simulink model "autopilota_v_15_last"  (R2020b)
settings: Solver=ode4  StartTime=0.0  StopTime=300  FixedStep=0.02  RelTol=1e-3
values from neighbouring files (symbols this model uses):
  attuatore_Amax = 20*(pi/180)    (= 0.349065850399)    [v2021_10_27_avvioSITL.m]    (also in v2021_10_27_calcoloAerodinamica.m)
  attuatore_Amin = -20*(pi/180)    (= -0.349065850399)    [v2021_10_27_avvioSITL.m]
  attuatore_Emax = 25*(pi/180)    (= 0.436332312999)    [v2021_10_27_avvioSITL.m]    (also in v2021_10_27_calcoloAerodinamica.m)
  attuatore_Emin = -25*(pi/180)    (= -0.436332312999)    [v2021_10_27_avvioSITL.m]
  attuatore_Rmax = 25*(pi/180)    (= 0.436332312999)    [v2021_10_27_avvioSITL.m]    (also in v2021_10_27_calcoloAerodinamica.m)
  attuatore_Rmin = -25*(pi/180)    (= -0.436332312999)    [v2021_10_27_avvioSITL.m]
  attuatore_Tmax = 0.99    [v2021_10_27_avvioSITL.m]
  attuatore_Tmin = 0    [v2021_10_27_avvioSITL.m]
  bias = [baccxINI,baccyINI,bacczINI,bpINI,bqINI,brINI]    [v2021_10_27_avvioSITL.m]
  final_h = 35    [v2021_10_27_avvioSITL.m]
  interventoA_05 = 20*0.8    (= 16)    [v2021_10_27_avvioSITL.m]
  interventoA_1 = 10    [v2021_10_27_avvioSITL.m]
  interventoE_05 = 25*0.8    (= 20)    [v2021_10_27_avvioSITL.m]
  interventoE_1 = 10    [v2021_10_27_avvioSITL.m]
  interventoT = 1*0.6    (= 0.6)    [v2021_10_27_avvioSITL.m]
  inv_A = 1    [v2021_10_27_avvioSITL.m]
  inv_comp_h = 1    [v2021_10_27_avvioSITL.m]
  inv_E = 1    [v2021_10_27_avvioSITL.m]
  inv_R = 1    [v2021_10_27_avvioSITL.m]
  inv_T = 1    [v2021_10_27_avvioSITL.m]
  K_AW_B_AP_quota = 1000    [v2021_10_27_avvioSITL.m]
  K_AW_B_becc = -250    [v2021_10_27_avvioSITL.m]
  K_AW_B_imb = 0    [v2021_10_27_avvioSITL.m]
  K_AW_B_roll = 500    [v2021_10_27_avvioSITL.m]
  K_imb_inv = -0.001306    [v2021_10_27_avvioSITL.m]
  Kd_AP_rotta = 0.995    [v2021_10_27_avvioSITL.m]
  Kd_h_app = 0.085    [v2021_10_27_avvioSITL.m]
  Kd_h_flare = 0.01    [v2021_10_27_avvioSITL.m]
  Ki_AP_quota_select = 0.01936    [v2021_10_27_avvioSITL.m]
  Ki_AP_rotta = 0.002    [v2021_10_27_avvioSITL.m]
  Ki_AP_vel = 0.025175    [v2021_10_27_avvioSITL.m]
  Ki_becch = -0.1963    [v2021_10_27_avvioSITL.m]
  Ki_h_app = 0.055    [v2021_10_27_avvioSITL.m]
  Ki_h_cruise = 0.008    [v2021_10_27_avvioSITL.m]
  Ki_h_flare = 0.07    [v2021_10_27_avvioSITL.m]
  Ki_roll = 0.004528    [v2021_10_27_avvioSITL.m]
  Kp_AP_quota_hold_h = 0.5503    [v2021_10_27_avvioSITL.m]
  Kp_AP_quota_hold_l = 0.5503    [v2021_10_27_avvioSITL.m]
  Kp_AP_quota_select = 0.02647    [v2021_10_27_avvioSITL.m]
  Kp_AP_rotta = 0.520    (= 0.52)    [v2021_10_27_avvioSITL.m]
  Kp_AP_vel = 0.132175    [v2021_10_27_avvioSITL.m]
  Kp_becch = -0.30    (= -0.3)    [v2021_10_27_avvioSITL.m]
  Kp_comp_h = 0.035    [v2021_10_27_avvioSITL.m]
  Kp_h_app_max = 0.086    [v2021_10_27_avvioSITL.m]
  Kp_h_app_min = 0.01    [v2021_10_27_avvioSITL.m]
  Kp_h_cruise = 0.04    [v2021_10_27_avvioSITL.m]
  Kp_h_flare = 0.1    [v2021_10_27_avvioSITL.m]
  Kp_imb = 0.0019415    [v2021_10_27_avvioSITL.m]
  Kp_p = 0.006913    [v2021_10_27_avvioSITL.m]
  Kp_q = -0.025    [v2021_10_27_avvioSITL.m]
  Kp_roll = 0.0718    [v2021_10_27_avvioSITL.m]
  Kp_Rotta_ATO = 4    [v2021_10_27_avvioSITL.m]
  Kp_Rotta_psi = -0.01    [v2021_10_27_avvioSITL.m]
  Q1B = [    2e-15;     2e-15 ... (first row only)    [COV_F1B.m]
  R1B = [     2e-14;             2e-14 ... (first row only)    [COV_F1B.m]
  safe_phi = 55    [v2021_10_27_avvioSITL.m]
  safe_V = 40    [v2021_10_27_avvioSITL.m]
  Sensor_Offsets = [0,0,0]    [v2021_10_27_avvioSITL.m]
  T_cal = 0.4    [v2021_10_27_avvioSITL.m]
  theta_rot = 10    [v2021_10_27_avvioSITL.m]
  time_alarm_SAFE = 300    [v2021_10_27_avvioSITL.m]
  tsamp = 0.02    [v2021_10_27_avvioSITL.m]
  update = [2,2,2]    [v2021_10_27_avvioSITL.m]
  V_max = 35    [v2021_10_27_avvioSITL.m]
  V_stall = 15    [v2021_10_27_avvioSITL.m]
  vd_ini = 0    [v2021_10_27_avvioSITL.m]
  vel_wp1_al = 25    [v2021_10_27_avvioSITL.m]
  vel_wp2_al = 20    [v2021_10_27_avvioSITL.m]
undefined symbols (not defined in the file or in its folder): DiscIntNeverNeededParam, Newton, Raphson, t_AP
libraries: simulink_extras x41, pid_lib x8, dspsigops x4, simulink x3, aerolibtransform2sys x2, aerolibtransform2 x2, cstblocks x1, aerosimlib x1
(part 1 of 11)
settings Model: Creator=39339  LastModifiedBy=39334
settings DataIOCC: ReturnWorkspaceOutputs=off
settings DebuggingCC: ParameterPrecisionLossMsg=none  ArithmeticOperatorsInVariantConditions=warning
settings ModelReferenceCC: ModelReferenceNumInstancesAllowed=Single
settings SFSimCC: SimUseLocalCustomCode=off  CustomCodeUndefinedFunction=UseInterfaceOnly
settings RTWCC: RTWUseLocalCustomCode=off
settings CodeAppCC: StateflowObjectComments=on

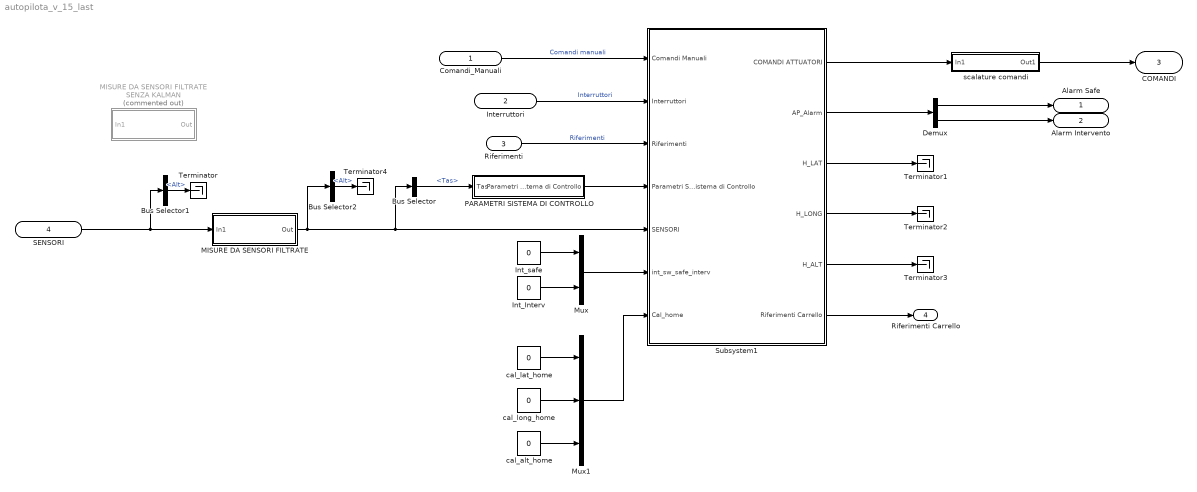
== system autopilota_v_15_last ==
  Comandi_Manuali : Inport  OutDataTypeStr=Bus: slBus4_manuali  SampleTime=[0.02,0]
  "Interruttori " : Inport  Port=2  OutDataTypeStr=Bus: slBus5_Interruttori  SampleTime=[0.02,0]
  Riferimenti : Inport  Port=3  OutDataTypeStr=Bus: slBus6_Riferimenti  SampleTime=[0.02,0]
  SENSORI : Inport  Port=4  OutDataTypeStr=Bus: slBus8_sensori2  SampleTime=[0.02,0]
  Bus Selector : BusSelector  OutputSignals=Tas
  Bus Selector1 : BusSelector  OutputSignals=Alt
  Bus Selector2 : BusSelector  OutputSignals=Alt
  Demux : Demux  Outputs=2
  Int_Interv : Constant  Value=0  SampleTime=t_AP
  Int_safe : Constant  Value=0  SampleTime=t_AP
  MISURE DA SENSORI FILTRATE : Subsystem
  MISURE DA SENSORI FILTRATE SENZA KALMAN : Subsystem  Commented=on
  Mux : Mux  Inputs=2
  Mux1 : Mux  Inputs=3
  PARAMETRI SISTEMA DI CONTROLLO : Subsystem
  Subsystem1 : Subsystem
  Terminator{,1..4} (5 alike) : Terminator
  cal_alt_home : Constant  Value=0  SampleTime=t_AP
  cal_lat_home : Constant  Value=0  SampleTime=t_AP
  cal_long_home : Constant  Value=0  SampleTime=t_AP
  "scalature comandi " : Subsystem
  Alarm Safe : Outport  OutDataTypeStr=double  PortDimensions=1  SampleTime=[0.02,0]  VectorParamsAs1DForOutWhenUnconnected=off
  Alarm Intervento : Outport  Port=2  OutDataTypeStr=double  PortDimensions=1  SampleTime=[0.02,0]  VectorParamsAs1DForOutWhenUnconnected=off
  "COMANDI " : Outport  Port=3  OutDataTypeStr=Bus: slBus8_comandi  SampleTime=[0.02,0]  VectorParamsAs1DForOutWhenUnconnected=off  LockScale=on
  Riferimenti Carrello : Outport  Port=4  VectorParamsAs1DForOutWhenUnconnected=off
  wires:
  cal_long_home/1 -> Mux1/2
  Comandi_Manuali/1 -> Subsystem1/1(Comandi Manuali)  "Comandi manuali"
  Bus Selector/1 -> PARAMETRI SISTEMA DI CONTROLLO/1(Tas)  "<Tas>"
  "Interruttori "/1 -> Subsystem1/2("Interruttori ")  "Interruttori"
  PARAMETRI SISTEMA DI CONTROLLO/1(Parametri Sistema di Controllo) -> Subsystem1/4(Parametri Sistema di Controllo)
  Subsystem1/3(H_LAT) -> Terminator1/1
  Demux/1 -> Alarm Safe/1
  Subsystem1/5(H_ALT) -> Terminator3/1
  cal_lat_home/1 -> Mux1/1
  Int_safe/1 -> Mux/1
  Riferimenti/1 -> Subsystem1/3(Riferimenti)  "Riferimenti"
  Mux1/1 -> Subsystem1/7(Cal_home)
  cal_alt_home/1 -> Mux1/3
  Int_Interv/1 -> Mux/2
  Demux/2 -> Alarm Intervento/1
  Subsystem1/4(H_LONG) -> Terminator2/1
  Subsystem1/2(AP_Alarm) -> Demux/1
  Mux/1 -> Subsystem1/6(int_sw_safe_interv)
  SENSORI/1 -> Bus Selector1/1, MISURE DA SENSORI FILTRATE/1(In1)
  MISURE DA SENSORI FILTRATE/1(Out) -> Bus Selector/1, Subsystem1/5(SENSORI), Bus Selector2/1
  "scalature comandi "/1(Out1) -> "COMANDI "/1
  Bus Selector2/1 -> Terminator4/1  "<Alt>"
  Bus Selector1/1 -> Terminator/1  "<Alt>"
  Subsystem1/6(Riferimenti Carrello) -> Riferimenti Carrello/1
  Subsystem1/1(COMANDI ATTUATORI) -> "scalature comandi "/1(In1)

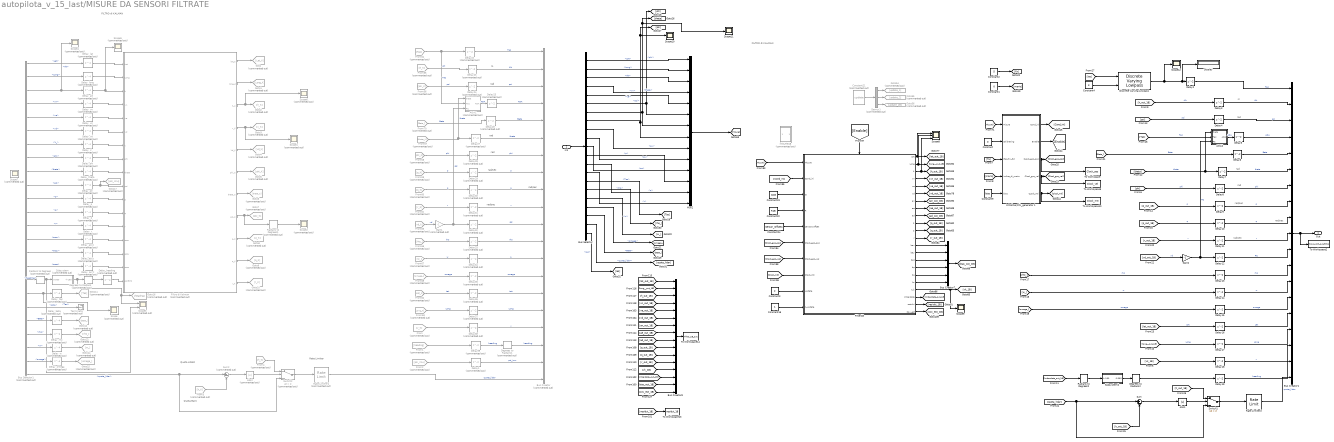
== system autopilota_v_15_last/MISURE DA SENSORI FILTRATE ==
  note: FILTRO di KALMAN
  note: m
  note: rad/sec
  note: rad/sec
  note: rad/sec
  note: rad
  note: rad
  note: rad
  note: Rate Limiter
  note: Quota Baro
  note: Quota LIDAR
  note: rad/sec
  note: rad/sec
  note: rad
  note: rad/sec
  note: FILTRO di KALMAN
  note: m
  note: rad
  note: rad
  In1 : Inport
  AOA1 : Subsystem  Commented=on
  AOA2 : Subsystem
  Abs1 : Abs
  Abs2 : Abs  Commented=on
  Bus Creator : BusCreator  Commented=on  Inputs=20  OutDataTypeStr=Bus: slBus7_sensori
  Bus Creator1 : BusCreator  Inputs=19  OutDataTypeStr=Bus: slBus7_sensori
  Bus Creator7 : BusCreator  Inputs=6
  Bus Creator8 : BusCreator  Inputs=16
  Bus Selector : BusSelector  OutputSignals=Lat,Long,Alt,vn,ve,phi,theta,psi,ax,ay,az,p,q,r,Tas,rho,w,omega,Beta,quota_lidar,Ias
  Bus Selector1 : BusSelector  Commented=on  OutputSignals=Lat,Long,Alt,vn,ve,vd,V_,phi,theta,psi,p,q,r,accx,accy,accz,heading,Tas,AOA,Beta,rho,w,omega,quota_lidar
  Constant : Constant  Value=0
  Constant1 : Constant  Value=0
  Constant16 : Constant
  Constant2 : Constant  Value=5
  Constant21 : Constant  Commented=on  Value=update
  Constant22 : Constant  Value=R1B
  Constant23 : Constant  Value=Q1B
  Constant24 : Constant  Value=Sensor_Offsets
  Constant3 : Constant  Value=2
  Constant4 : Constant  Value=3
  Constant9 : Constant  Value=bias
  Degrees to Radians : simulink_extras/Transformations/Degrees to Radians  Commented=on
  Degrees to Radians1 : simulink_extras/Transformations/Degrees to Radians  Commented=on
  Degrees to Radians2 : simulink_extras/Transformations/Degrees to Radians
  Delay{1,22..39} (19 alike) : Delay  Commented=on
  Delay{2..19} (18 alike) : Delay
  Delay_V_ : Delay  Commented=on  DelayLength=4
  Delay_accx : Delay  Commented=on  DelayLength=4
  Delay_accy : Delay  Commented=on  DelayLength=4
  Delay_accz : Delay  Commented=on  DelayLength=4
  Delay_alt : Delay  Commented=on  DelayLength=4
  Delay_beta : Delay  Commented=on  DelayLength=4
  Delay_heading : Delay  Commented=on  DelayLength=4
  Delay_lat : Delay  Commented=on  DelayLength=4
  Delay_long : Delay  Commented=on  DelayLength=4
  Delay_omega : Delay  Commented=on  DelayLength=4
  Delay_p : Delay  Commented=on  DelayLength=4
  Delay_phi : Delay  Commented=on  DelayLength=4
  Delay_psi : Delay  Commented=on  DelayLength=4
  Delay_q : Delay  Commented=on  DelayLength=4
  Delay_r : Delay  Commented=on  DelayLength=4
  Delay_rho : Delay  Commented=on  DelayLength=4
  Delay_tas : Delay  Commented=on  DelayLength=4
  Delay_theta : Delay  Commented=on  DelayLength=4
  Delay_vd : Delay  Commented=on  DelayLength=4
  Delay_ve : Delay  Commented=on  DelayLength=4
  Delay_vn : Delay  Commented=on  DelayLength=4
  Delay_w : Delay  Commented=on  DelayLength=4
  Demux1 : Demux  Commented=on  Outputs=3
  Discrete Varying Lowpass : cstblocks/Linear Parameter Varying/Discrete Varying Lowpass  N=2  w0=0  Ts=0.02
      settings: SourceProductBaseCode=CT
  Display : Display
  Filter1B : Subsystem
  Filtro di Kalman : Subsystem  Commented=on
  From : From  Commented=on  GotoTag=v_K
  From1 : From  Commented=on  GotoTag=heading
  From2 : From  Commented=on  GotoTag=psi_imu
  From3 : From  Commented=on  GotoTag=h_K
  From4 : From  Commented=on  GotoTag=h_K
  From55 : From  Commented=on  GotoTag=h_K
  From56 : From  Commented=on  GotoTag=psi_K
  From57 : From  Commented=on  GotoTag=theta_K
  From58 : From  Commented=on  GotoTag=phi_K
  From59 : From  Commented=on  GotoTag=p_K
  From60 : From  Commented=on  GotoTag=q_K
  From61 : From  Commented=on  GotoTag=r_K
  From62 : From  Commented=on  GotoTag=Lat_K
  From63 : From  Commented=on  GotoTag=Long_K
  From64 : From  Commented=on  GotoTag=Tas
  From65 : From  Commented=on  GotoTag=vd_k
  From66 : From  Commented=on  GotoTag=rho_
  From67 : From  Commented=on  GotoTag=w_
  From68 : From  Commented=on  GotoTag=omega_
  From70 : From  Commented=on  GotoTag=Beta_
  Gain1 : Gain  Commented=on  Gain=-1
  Gain2 : Gain  Gain=-1
  Goto : Goto  Commented=on  GotoTag=Lat_K
  Goto1 : Goto  Commented=on  GotoTag=Long_K
  Goto10 : Goto  Commented=on  GotoTag=r_K
  Goto11 : Goto  Commented=on  GotoTag=Tas
  Goto12 : Goto  Commented=on  GotoTag=Beta_
  Goto13 : Goto  Commented=on  GotoTag=rho_
  Goto14 : Goto  Commented=on  GotoTag=w_
  Goto15 : Goto  Commented=on  GotoTag=omega_
  Goto16 : Goto  Commented=on  GotoTag=heading
  Goto17 : Goto  Commented=on  GotoTag=psi_imu
  Goto2 : Goto  Commented=on  GotoTag=h_K
  Goto3 : Goto  Commented=on  GotoTag=v_K
  Goto4 : Goto  Commented=on  GotoTag=vd_k
  Goto5 : Goto  Commented=on  GotoTag=phi_K
  Goto54 : Goto  Commented=on  GotoTag=update_1
  Goto55 : Goto  Commented=on  GotoTag=update_2
  Goto56 : Goto  Commented=on  GotoTag=update_2B
  Goto6 : Goto  Commented=on  GotoTag=theta_K
  Goto7 : Goto  Commented=on  GotoTag=psi_K
  Goto8 : Goto  Commented=on  GotoTag=p_K
  Goto9 : Goto  Commented=on  GotoTag=q_K
  MISURE1B : Subsystem  Commented=on
  Mux2 : Mux  Inputs=14
  Radians to Degrees : simulink_extras/Transformations/Radians to Degrees  Commented=on
  Radians to Degrees1 : simulink_extras/Transformations/Radians to Degrees  Commented=on
  Radians to Degrees2 : simulink_extras/Transformations/Radians to Degrees
  Rate Limiter1 : RateLimiter  Commented=on  RisingSlewLimit=6  FallingSlewLimit=-6  SampleTimeMode=inherited
  Rate Limiter2 : RateLimiter  RisingSlewLimit=6  FallingSlewLimit=-6  SampleTimeMode=inherited
  Scope{,1..2,4..7} (7 alike) : Scope  Commented=on
  Scope{9..12} (4 alike) : Scope
  Scope3 : Scope  Commented=on  NumInputPorts=2
  Scope8 : Scope  NumInputPorts=3
  Subsystem : Subsystem  Commented=on
  Subsystem2 : Subsystem
  Sum : Sum  Inputs=|+-
  Sum2 : Sum  Commented=on  Inputs=|+-
  Switch1 : Switch  Criteria=u2 > Threshold  Threshold=2
  Switch2 : Switch  Commented=on  Criteria=u2 > Threshold  Threshold=2
  Terminator : Terminator  Commented=on
  To Workspace : ToWorkspace  VariableName=Clock_pos  SaveFormat=Timeseries  SampleTime=-1
  To Workspace10 : ToWorkspace  VariableName=Clock_mti  SaveFormat=Timeseries  SampleTime=-1
  To Workspace13 : ToWorkspace  VariableName=residui_1B  SaveFormat=Structure With Time  SampleTime=-1
  To Workspace14 : ToWorkspace  VariableName=Filtro_1B_out  SaveFormat=Timeseries  SampleTime=-1
  To Workspace2 : ToWorkspace  VariableName=Prova_WP_out_filtro  SaveFormat=Timeseries  SampleTime=-1
  To Workspace9 : ToWorkspace  VariableName=Clock_vel  SaveFormat=Timeseries  SampleTime=-1
  initializer/Clk_generator 1 : Subsystem
  Out : Outport  OutDataTypeStr=Bus: slBus7_sensori  VectorParamsAs1DForOutWhenUnconnected=off
  wires:
  Bus Selector1/1 -> Delay_lat/1  "<Lat>"
  Bus Selector1/23 -> Delay_omega/1  "<omega>"
  Bus Selector1/2 -> Delay_long/1  "<Long>"
  Bus Selector1/3 -> Scope4/1, Delay_alt/1  "<Alt>"
  Bus Selector1/4 -> Delay_vn/1  "<vn>"
  Bus Selector1/5 -> Delay_ve/1  "<ve>"
  Bus Selector1/6 -> Delay_vd/1  "<vd>"
  Bus Selector1/7 -> Delay_V_/1  "<V_>"
  Bus Selector1/8 -> Delay_phi/1  "<phi>"
  Bus Selector1/9 -> Delay_theta/1  "<theta>"
  Bus Selector1/10 -> Delay_psi/1  "<psi>"
  Bus Selector1/11 -> Delay_p/1  "<p>"
  Bus Selector1/12 -> Delay_q/1  "<q>"
  Bus Selector1/13 -> Delay_r/1  "<r>"
  Bus Selector1/14 -> Delay_accx/1  "<accx>"
  Bus Selector1/15 -> Delay_accy/1  "<accy>"
  Bus Selector1/16 -> Delay_accz/1  "<accz>"
  Bus Selector1/17 -> Radians to Degrees/1  "<heading>"
  Filtro di Kalman/1(lat_K) -> Goto/1
  Filtro di Kalman/2(long_K) -> Goto1/1
  Filtro di Kalman/3(h_K) -> Scope6/1, Goto2/1
  Filtro di Kalman/4(v_K) -> Scope1/1, Goto3/1
  Filtro di Kalman/6(phi_K) -> Goto5/1
  Filtro di Kalman/7(theta_K) -> Goto6/1
  Filtro di Kalman/9(p_K) -> Goto8/1
  Filtro di Kalman/11(r_K) -> Goto10/1
  Filtro di Kalman/10(q_K) -> Goto9/1
  Bus Selector1/18 -> Scope/1, Delay_tas/1  "<Tas>"
  Bus Selector1/19 -> Terminator/1  "<AOA>"
  Bus Selector1/20 -> Delay_beta/1  "<Beta>"
  Bus Selector1/21 -> Delay_rho/1  "<rho>"
  Bus Selector1/22 -> Delay_w/1  "<w>"
  From55/1 -> Delay23/1  "Alt"
  From56/1 -> Delay24/1  "psi"
  From57/1 -> AOA1/1(theta), Delay27/1  "theta"
  From58/1 -> Delay28/1  "phi"
  From59/1 -> Delay29/1  "p"
  From60/1 -> Delay30/1  "q"
  From61/1 -> Delay31/1  "r"
  From63/1 -> Delay37/1  "Long"
  From64/1 -> AOA1/2(Tas), Delay22/1  "Tas"
  From65/1 -> Gain1/1  "vd"
  From66/1 -> Delay33/1  "rho"
  From67/1 -> Delay34/1  "w"
  From68/1 -> Delay35/1  "omega"
  AOA1/1(AOA) -> Delay25/1  "AOA"
  From70/1 -> Delay26/1  "Beta"
  From62/1 -> Delay36/1  "Lat"
  Gain1/1 -> AOA1/3(RC), Delay32/1  "RC"
  Filtro di Kalman/5(Vd_K) -> Goto4/1
  Delay_lat/1 -> Filtro di Kalman/1("Lat ")
  Delay_long/1 -> Filtro di Kalman/2("Long ")
  Delay_psi/1 -> Goto17/1, Filtro di Kalman/10(psi)
  Delay_p/1 -> Filtro di Kalman/11(p)
  Delay_q/1 -> Filtro di Kalman/12(q)
  Delay_r/1 -> Filtro di Kalman/13(r)
  Delay_accx/1 -> Filtro di Kalman/14(accx)
  Delay_accy/1 -> Filtro di Kalman/15(accy)
  Delay_accz/1 -> Filtro di Kalman/16(accz)
  Delay_vd/1 -> Filtro di Kalman/6(vd)
  Delay_V_/1 -> Filtro di Kalman/7("v ")
  Delay_theta/1 -> Filtro di Kalman/9(theta)
  Delay_ve/1 -> Filtro di Kalman/5("ve ")
  Delay_vn/1 -> Filtro di Kalman/4(vn)
  Delay_alt/1 -> Scope5/1, Filtro di Kalman/3(h)
  Delay_phi/1 -> Filtro di Kalman/8(phi)
  Delay_tas/1 -> Goto11/1
  Delay_beta/1 -> Goto12/1
  Delay_rho/1 -> Goto13/1
  Delay_w/1 -> Goto14/1
  Delay_omega/1 -> Goto15/1
  Filtro di Kalman/8(psi_K) -> Radians to Degrees1/1, Goto7/1
  Radians to Degrees1/1 -> Scope2/1
  Delay22/1 -> Bus Creator/1  "Tas"
  Delay23/1 -> Bus Creator/2  "Alt"
  Delay24/1 -> Bus Creator/3  "psi"
  Delay25/1 -> Bus Creator/4  "AOA"
  Delay26/1 -> Bus Creator/5  "Beta"
  Delay27/1 -> Bus Creator/6  "theta"
  Delay28/1 -> Bus Creator/7  "phi"
  Delay29/1 -> Bus Creator/8  "p"
  Delay30/1 -> Bus Creator/9  "q"
  Delay31/1 -> Bus Creator/10  "r"
  Delay32/1 -> Bus Creator/11  "RC"
  Delay33/1 -> Bus Creator/12  "rho"
  Delay34/1 -> Bus Creator/13  "w"
  Delay35/1 -> Bus Creator/14  "omega"
  Delay36/1 -> Bus Creator/15  "Lat"
  Delay37/1 -> Bus Creator/16  "Long"
  Subsystem/1("+-180 ") -> Degrees to Radians/1, Scope3/1, Goto16/1
  Radians to Degrees/1 -> Scope3/2, Subsystem/1(0-360)
  Delay_heading/1 -> Filtro di Kalman/17(psiGPS)
  Degrees to Radians/1 -> Delay_heading/1
  Delay38/1 -> Bus Creator/17  "v"
  From/1 -> Delay38/1
  From1/1 -> Delay39/1
  Delay39/1 -> Degrees to Radians1/1  "heading"
  From2/1 -> Delay1/1
  Delay1/1 -> Bus Creator/19  "psi_imu"
  Bus Selector1/24 -> Switch2/3, Sum2/1  "<quota_lidar>"
  Abs2/1 -> Switch2/2
  Switch2/1 -> Rate Limiter1/1
  From3/1 -> Sum2/2
  From4/1 -> Switch2/1
  Rate Limiter1/1 -> Bus Creator/20  "quota_lidar"
  Sum2/1 -> Abs2/1
  Degrees to Radians1/1 -> Bus Creator/18  "heading"
  Constant16/1 -> Filter1B/10(k_update)
  [Misure] -> initializer/Clk_generator 1/1(Misure)
  Delay14/1 -> Bus Creator1/13  "w"
  [Clock_gps_vel] -> Filter1B/7(Clock_gps_vel)
  Filter1B/21(residui) -> [residui_1B]
  Bus Selector/14 -> Mux2/14  "<r>"
  Filter1B/11(q) -> [q_out_1B]
  Filter1B/9(ad) -> [ad_out_1B]
  Filter1B/16(bp) -> Bus Creator7/4
  Gain2/1 -> AOA2/3(RC), Delay12/1  "RC"
  Filter1B/17(bq) -> Bus Creator7/5
  [long__out_1B] -> Bus Creator8/2
  [Clock_mti] -> Filter1B/8(Clock_mti)
  [mario] -> initializer/Clk_generator 1/4(indice_di_mario)
  Bus Creator7/1 -> [bias_out_1B]
  [h_out_1B] -> Bus Creator8/3
  [an_out_1B] -> Bus Creator8/7
  [Clock_gps_pos] -> Filter1B/6(Clock_gps_pos)
  Bus Selector/10 -> Mux2/10  "<ay>"
  [ad_out_1B] -> Bus Creator8/9
  Filter1B/5(ve) -> [ve_out_1B]
  Filter1B/3(h) -> Scope8/3, [h_out_1B]
  [ae_out_1B] -> Bus Creator8/8
  Bus Creator8/1 -> To Workspace14/1
  Bus Selector/13 -> Mux2/13  "<q>"
  Constant3/1 -> Filter1B/9(update)
  [h_out_1B] -> Delay3/1  "Alt"
  Constant9/1 -> initializer/Clk_generator 1/5(bias)
  Filter1B/4(vn) -> [vn_out_1B]
  [lat_out_1B] -> Delay16/1  "Lat"
  [w_] -> Delay14/1  "w"
  Constant24/1 -> Filter1B/5(sensors offset)
  [Cond_ini] -> Filter1B/2(Cond_ini)
  Constant2/1 -> [fix]
  Filter1B/13(bax) -> Bus Creator7/1
  Filter1B/8(ae) -> [ae_out_1B]
  Filter1B/15(baz) -> Bus Creator7/3
  Delay19/1 -> Bus Creator1/18  "heading"
  [Misure] -> Filter1B/1(Misure)
  Delay9/1 -> Bus Creator1/8  "p"
  Filter1B/12(r) -> [r_out_1B]
  [vd_out_1B] -> Gain2/1  "vd"
  Filter1B/10(p) -> [p_out_1B]
  [cov_est_1B] -> Bus Creator8/16
  initializer/Clk_generator 1/5(CLock_mti) -> To Workspace10/1, [Clock_mti]
  Filter1B/6(vd) -> [vd_out_1B]
  Filter1B/22(Cov_est) -> [cov_est_1B]
  [vk_1B] -> Delay18/1
  initializer/Clk_generator 1/2(Enable) -> [Enable]
  [vn_out_1B] -> Bus Creator8/4
  [imbardata_out_1B] -> Bus Creator8/14
  [vd_out_1B] -> Bus Creator8/6
  [Beta_] -> Delay6/1  "Beta"
  Delay6/1 -> Bus Creator1/5  "Beta"
  [rho_] -> Delay13/1  "rho"
  Demux1/2 -> Goto55/1
  Mux2/1 -> [Misure]
  Demux1/1 -> Goto54/1
  initializer/Clk_generator 1/4("Clock_gps_vel ") -> To Workspace9/1, [Clock_gps_vel]
  Delay4/1 -> Bus Creator1/3  "psi"
  [bias_out_1B] -> Bus Creator8/15
  Filter1B/18(br) -> Bus Creator7/6
  [ve_out_1B] -> Bus Creator8/5
  Constant/1 -> initializer/Clk_generator 1/2(calibrating)
  initializer/Clk_generator 1/3(CLock_gps_pos) -> To Workspace/1, [Clock_gps_pos]
  Delay15/1 -> Bus Creator1/14  "omega"
  Constant22/1 -> Filter1B/4(R)
  [p_out_1B] -> Delay9/1  "p"
  [phi] -> Delay8/1  "phi"
  Filter1B/2(Long) -> [long__out_1B], Scope8/2
  Bus Selector/5 -> Mux2/5  "<ve>"
  [lat_out_1B] -> Bus Creator8/1
  Bus Selector/15 -> [Tas]  "<Tas>"
  Delay18/1 -> Bus Creator1/17  "v"
  [q_out_1B] -> Bus Creator8/11
  Bus Selector/1 -> Mux2/1  "<Lat>"
  initializer/Clk_generator 1/1(Cond_ini) -> [Cond_ini]
  [fix] -> initializer/Clk_generator 1/3(Gps_fix_3d)
  Bus Selector/3 -> Mux2/3  "<Alt>"
  Constant21/1 -> Demux1/1
  [p_out_1B] -> Bus Creator8/10
  Bus Selector/7 -> Scope11/1, [theta], Mux2/7  "<theta>"
  [vk_1B] -> Bus Creator8/13
  Delay8/1 -> Bus Creator1/7  "phi"
  Filter1B/14(bay) -> Bus Creator7/2
  Delay12/1 -> Bus Creator1/11  "RC"
  Bus Creator1/1 -> To Workspace2/1, Out/1
  Delay5/1 -> Bus Creator1/4  "AOA"
  Constant1/1 -> [mario]
  Delay17/1 -> Bus Creator1/16  "Long"
  Constant23/1 -> Filter1B/3(Q)
  [r_out_1B] -> Delay11/1  "r"
  Bus Selector/8 -> Scope10/1, [psi], Mux2/8  "<psi>"
  Delay16/1 -> Bus Creator1/15  "Lat"
  [q_out_1B] -> Delay10/1  "q"
  Delay11/1 -> Bus Creator1/10  "r"
  [Tas] -> AOA2/2(Tas)  "Tas"
  [long__out_1B] -> Delay17/1  "Long"
  [Enable] -> Filter1B/Enable
  [imbardata_out_1B] -> Radians to Degrees2/1
  Demux1/3 -> Goto56/1
  Filter1B/20(Imbardata) -> [imbardata_out_1B]
  Delay13/1 -> Bus Creator1/12  "rho"
  Filter1B/1(Lat) -> Scope8/1, [lat_out_1B]
  Delay10/1 -> Bus Creator1/9  "q"
  Delay7/1 -> Bus Creator1/6  "theta"
  Delay3/1 -> Bus Creator1/2  "Alt"
  Filter1B/7(an) -> [an_out_1B]
  [omega_] -> Delay15/1  "omega"
  [theta] -> AOA2/1(theta), Delay7/1  "theta"
  Delay2/1 -> Bus Creator1/1  "Tas"
  AOA2/1(AOA) -> Delay5/1  "AOA"
  [residui_1B] -> To Workspace13/1
  [psi] -> Delay4/1  "psi"
  [r_out_1B] -> Bus Creator8/12
  [quota_lidar] -> Switch1/3, Sum/1
  [h_out_1B] -> Sum/2
  Sum/1 -> Abs1/1
  Abs1/1 -> Switch1/2
  [h_out_1B] -> Switch1/1
  Switch1/1 -> Rate Limiter2/1
  Rate Limiter2/1 -> Bus Creator1/19  "quota_lidar"
  In1/1 -> Bus Selector/1
  Bus Selector/2 -> Mux2/2  "<Long>"
  Bus Selector/4 -> Mux2/4  "<vn>"
  Bus Selector/6 -> [phi], Mux2/6  "<phi>"
  Bus Selector/9 -> Mux2/9  "<ax>"
  Bus Selector/11 -> Mux2/11  "<az>"
  Bus Selector/12 -> Mux2/12  "<p>"
  Bus Selector/16 -> [rho_]  "<rho>"
  Bus Selector/17 -> [w_]  "<w>"
  Bus Selector/18 -> [omega_]  "<omega>"
  Bus Selector/19 -> [Beta_]  "<Beta>"
  Bus Selector/20 -> [quota_lidar]  "<quota_lidar>"
  Filter1B/19(V_k) -> Scope9/1, [vk_1B]
  Degrees to Radians2/1 -> Delay19/1
  Radians to Degrees2/1 -> Subsystem2/1(+-180)
  Subsystem2/1(0-360) -> Degrees to Radians2/1
  Bus Selector/21 -> [Ias]  "<Ias>"
  [Ias] -> Discrete Varying Lowpass/1
  Discrete Varying Lowpass/1 -> Display/1, Delay2/1, Scope12/1
  Constant4/1 -> Discrete Varying Lowpass/2

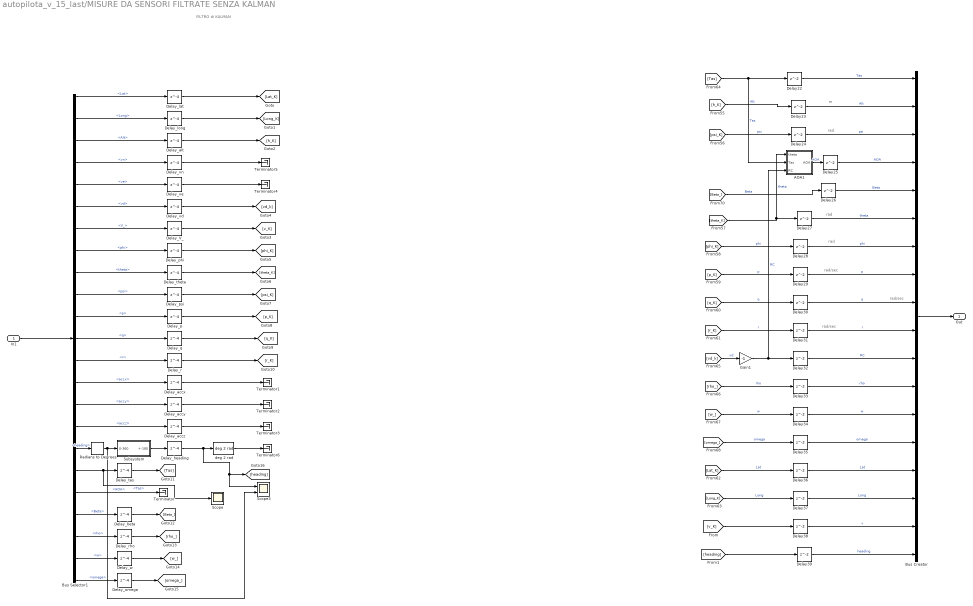
== system autopilota_v_15_last/MISURE DA SENSORI FILTRATE SENZA KALMAN ==
  note: rad
  note: rad
  note: rad
  note: rad/sec
  note: rad/sec
  note: rad/sec
  note: m
  note: FILTRO di KALMAN
  In1 : Inport
  AOA1 : Subsystem
  Bus Creator : BusCreator  Inputs=18  OutDataTypeStr=Bus: slBus7_sensori
  Bus Selector1 : BusSelector  OutputSignals=Lat,Long,Alt,vn,ve,vd,V_,phi,theta,psi,p,q,r,accx,accy,accz,heading,Tas,AOA,Beta,rho,w,omega
  Delay{22..39} (18 alike) : Delay
  Delay_V_ : Delay  DelayLength=4
  Delay_accx : Delay  DelayLength=4
  Delay_accy : Delay  DelayLength=4
  Delay_accz : Delay  DelayLength=4
  Delay_alt : Delay  DelayLength=4
  Delay_beta : Delay  DelayLength=4
  Delay_heading : Delay  DelayLength=4
  Delay_lat : Delay  DelayLength=4
  Delay_long : Delay  DelayLength=4
  Delay_omega : Delay  DelayLength=4
  Delay_p : Delay  DelayLength=4
  Delay_phi : Delay  DelayLength=4
  Delay_psi : Delay  DelayLength=4
  Delay_q : Delay  DelayLength=4
  Delay_r : Delay  DelayLength=4
  Delay_rho : Delay  DelayLength=4
  Delay_tas : Delay  DelayLength=4
  Delay_theta : Delay  DelayLength=4
  Delay_vd : Delay  DelayLength=4
  Delay_ve : Delay  DelayLength=4
  Delay_vn : Delay  DelayLength=4
  Delay_w : Delay  DelayLength=4
  Gain1 : Gain  Gain=-1
  Radians to Degrees : simulink_extras/Transformations/Radians to Degrees
  Scope : Scope
  Scope3 : Scope  NumInputPorts=2
  Subsystem : Subsystem
  Terminator{,1..6} (7 alike) : Terminator
  deg 2 rad : aerosimlib/Unit Conversion/Angular position/deg 2 rad
      settings: SourceProductName=AeroSim Blockset
  Out : Outport  OutDataTypeStr=Bus: slBus7_sensori  VectorParamsAs1DForOutWhenUnconnected=off
  wires:
  Delay39/1 -> Bus Creator/18  "heading"
  [heading] -> Delay39/1
  [v_K] -> Delay38/1
  Delay38/1 -> Bus Creator/17  "v"
  deg 2 rad/1 -> Terminator6/1
  Radians to Degrees/1 -> Subsystem/1(0-360), Scope3/2
  Subsystem/1("+-180 ") -> Delay_heading/1
  Delay37/1 -> Bus Creator/16  "Long"
  Delay36/1 -> Bus Creator/15  "Lat"
  Delay35/1 -> Bus Creator/14  "omega"
  Delay34/1 -> Bus Creator/13  "w"
  Delay33/1 -> Bus Creator/12  "rho"
  Delay32/1 -> Bus Creator/11  "RC"
  Delay31/1 -> Bus Creator/10  "r"
  Delay30/1 -> Bus Creator/9  "q"
  Delay29/1 -> Bus Creator/8  "p"
  Delay28/1 -> Bus Creator/7  "phi"
  Delay27/1 -> Bus Creator/6  "theta"
  Delay26/1 -> Bus Creator/5  "Beta"
  Delay25/1 -> Bus Creator/4  "AOA"
  Delay24/1 -> Bus Creator/3  "psi"
  Delay23/1 -> Bus Creator/2  "Alt"
  Delay22/1 -> Bus Creator/1  "Tas"
  Delay_psi/1 -> [psi_K]
  Delay_omega/1 -> [omega_]
  Delay_w/1 -> [w_]
  Delay_rho/1 -> [rho_]
  Delay_beta/1 -> [Beta_]
  Delay_tas/1 -> [Tas]
  Delay_ve/1 -> Terminator4/1
  Delay_V_/1 -> [v_K]
  Delay_accz/1 -> Terminator3/1
  Delay_accy/1 -> Terminator2/1
  Delay_accx/1 -> Terminator1/1
  Delay_vd/1 -> [vd_k]
  Gain1/1 -> Delay32/1, AOA1/3(RC)  "RC"
  [Lat_K] -> Delay36/1  "Lat"
  [Beta_] -> Delay26/1  "Beta"
  AOA1/1(AOA) -> Delay25/1  "AOA"
  [omega_] -> Delay35/1  "omega"
  [w_] -> Delay34/1  "w"
  [rho_] -> Delay33/1  "rho"
  [vd_k] -> Gain1/1  "vd"
  [Tas] -> Delay22/1, AOA1/2(Tas)  "Tas"
  [Long_K] -> Delay37/1  "Long"
  [r_K] -> Delay31/1  "r"
  [q_K] -> Delay30/1  "q"
  [p_K] -> Delay29/1  "p"
  [phi_K] -> Delay28/1  "phi"
  [theta_K] -> Delay27/1, AOA1/1(theta)  "theta"
  [psi_K] -> Delay24/1  "psi"
  [h_K] -> Delay23/1  "Alt"
  Bus Creator/1 -> Out/1
  Bus Selector1/22 -> Delay_w/1  "<w>"
  Bus Selector1/21 -> Delay_rho/1  "<rho>"
  Bus Selector1/20 -> Delay_beta/1  "<Beta>"
  Bus Selector1/19 -> Terminator/1  "<AOA>"
  Bus Selector1/18 -> Delay_tas/1, Scope/1  "<Tas>"
  Delay_q/1 -> [q_K]
  Delay_r/1 -> [r_K]
  Delay_p/1 -> [p_K]
  Delay_theta/1 -> [theta_K]
  Delay_phi/1 -> [phi_K]
  Delay_alt/1 -> [h_K]
  Delay_long/1 -> [Long_K]
  Delay_lat/1 -> [Lat_K]
  Bus Selector1/17 -> Radians to Degrees/1  "<heading>"
  Bus Selector1/16 -> Delay_accz/1  "<accz>"
  Bus Selector1/15 -> Delay_accy/1  "<accy>"
  Bus Selector1/14 -> Delay_accx/1  "<accx>"
  Bus Selector1/13 -> Delay_r/1  "<r>"
  Bus Selector1/12 -> Delay_q/1  "<q>"
  Bus Selector1/11 -> Delay_p/1  "<p>"
  Bus Selector1/10 -> Delay_psi/1  "<psi>"
  Bus Selector1/9 -> Delay_theta/1  "<theta>"
  Bus Selector1/8 -> Delay_phi/1  "<phi>"
  Bus Selector1/7 -> Delay_V_/1  "<V_>"
  Bus Selector1/6 -> Delay_vd/1  "<vd>"
  Bus Selector1/5 -> Delay_ve/1  "<ve>"
  Bus Selector1/4 -> Delay_vn/1  "<vn>"
  Bus Selector1/3 -> Delay_alt/1  "<Alt>"
  Bus Selector1/2 -> Delay_long/1  "<Long>"
  Bus Selector1/23 -> Delay_omega/1  "<omega>"
  Bus Selector1/1 -> Delay_lat/1  "<Lat>"
  In1/1 -> Bus Selector1/1
  Delay_vn/1 -> Terminator5/1
  Delay_heading/1 -> deg 2 rad/1, [heading], Scope3/1

== system autopilota_v_15_last/PARAMETRI SISTEMA DI CONTROLLO ==
  Tas : Inport
  Bus Creator1 : BusCreator  Inputs=19
  K AntiWindup-Bumpless AP quota : Constant  Value=K_AW_B_AP_quota  OutDataTypeStr=single  SampleTime=t_AP
  K AntiWindup-Bumpless controllore beccheggio : Constant  Value=K_AW_B_becc  OutDataTypeStr=single  SampleTime=t_AP
  K AntiWindup-Bumpless controllore imbardata : Constant  Value=K_AW_B_imb  OutDataTypeStr=single  SampleTime=t_AP
  K AntiWindup-Bumpless controllore rollio : Constant  Value=K_AW_B_roll  OutDataTypeStr=single  SampleTime=t_AP
  K AntiWindup-Bumpless controllore rollio1 : Constant  Commented=on  Value=500  OutDataTypeStr=int16
  K controllo imbardata inversa : Constant  Value=K_imb_inv  OutDataTypeStr=single  SampleTime=t_AP
  Ki AP quota Select : Constant  Value=Ki_AP_quota_select  OutDataTypeStr=single  SampleTime=t_AP
  Ki AP rotta1 : Constant  Value=Kd_AP_rotta  OutDataTypeStr=single  SampleTime=t_AP
  Ki AP velocità : Constant  Value=Ki_AP_vel  OutDataTypeStr=single  SampleTime=t_AP
  Ki controllore  beccheggio1 : Constant  Value=Ki_becch  OutDataTypeStr=single  SampleTime=t_AP
  Ki controllore  rollio1 : Constant  Commented=on  Value=0.013  OutDataTypeStr=single
  Ki controllore  rollio2 : Constant  Commented=on  Value=0.025  OutDataTypeStr=single
  Ki controllore  rollio3 : Constant  Value=Ki_roll  OutDataTypeStr=single  SampleTime=t_AP
  Kp AP quota Hold2 : Constant  Commented=on  Value=0.15  OutDataTypeStr=single
  Kp AP quota Select : Constant  Value=Kp_AP_quota_select  OutDataTypeStr=single  SampleTime=t_AP
  Kp AP rotta : Constant  Value=Kp_AP_rotta  OutDataTypeStr=single  SampleTime=t_AP
  Kp AP rotta1 : Constant  Commented=on  Value=0.3  OutDataTypeStr=single
  Kp AP velocità : Constant  Value=Kp_AP_vel  OutDataTypeStr=single  SampleTime=t_AP
  Kp controllore  rollio1 : Constant  Commented=on  Value=0.15  OutDataTypeStr=single
  Kp controllore  rollio2 : Constant  Commented=on  Value=0.13  OutDataTypeStr=single
  Kp controllore  rollio3 : Constant  Value=Kp_roll  OutDataTypeStr=single  SampleTime=t_AP
  Kp controllore  velocità rollio1 : Constant  Commented=on  Value=0.04  OutDataTypeStr=single
  Kp controllore  velocità rollio2 : Constant  Commented=on  Value=0.05  OutDataTypeStr=single
  Kp controllore  velocità rollio3 : Constant  Value=Kp_p  OutDataTypeStr=single  SampleTime=t_AP
  Kp controllore beccheggio1 : Constant  Value=Kp_becch  OutDataTypeStr=single  SampleTime=t_AP
  Kp controllore imbardata : Constant  Value=Kp_imb  OutDataTypeStr=single  SampleTime=t_AP
  Kp controllore imbardata1 : Constant  Commented=on  Value=-0.1  OutDataTypeStr=single
  Kp controllore velocità beccheggio1 : Constant  Value=Kp_q  OutDataTypeStr=single  SampleTime=t_AP
  Saturation : Saturate  UpperLimit=Kp_AP_quota_hold_h  LowerLimit=Kp_AP_quota_hold_l*0.9
  n-D Lookup Table : Lookup_n-D  NumberOfTableDimensions=1  BreakpointsForDimension1=[V_stall V_max*0.8]  Table=[Kp_AP_quota_hold_l Kp_AP_quota_hold_h]  RndMeth=Simplest  InputSameDT=on
  Parametri Sistema di Controllo : Outport  VectorParamsAs1DForOutWhenUnconnected=off
  wires:
  Bus Creator1/1 -> Parametri Sistema di Controllo/1  "Cond.Volo.Richiesta"
  Kp controllore imbardata/1 -> Bus Creator1/7  "Kp_imb"
  Kp AP velocità/1 -> Bus Creator1/8  "Kp_AP_vel"
  Saturation/1 -> Bus Creator1/10  "Kp_AP_quota_hold"
  Kp AP quota Select/1 -> Bus Creator1/11  "Kp_AP_quota_select"
  Ki AP quota Select/1 -> Bus Creator1/12  "Ki_AP_quota_select"
  Kp AP rotta/1 -> Bus Creator1/13  "Kp_AP_rotta"
  K AntiWindup-Bumpless controllore beccheggio/1 -> Bus Creator1/15  "K_AW-B_becc"
  K AntiWindup-Bumpless controllore rollio/1 -> Bus Creator1/16  "K_AW-B_roll"
  K AntiWindup-Bumpless controllore imbardata/1 -> Bus Creator1/17  "K_AW-B_imb"
  K AntiWindup-Bumpless AP quota/1 -> Bus Creator1/18  "K_AW-B_AP_quota"
  Ki AP velocità/1 -> Bus Creator1/9  "Ki_AP_vel"
  Ki AP rotta1/1 -> Bus Creator1/14  "Ki_AP_rotta"
  Kp controllore  rollio3/1 -> Bus Creator1/4  "Kp_roll"
  Kp controllore  velocità rollio3/1 -> Bus Creator1/6  "Kp_p"
  Ki controllore  rollio3/1 -> Bus Creator1/5  "Ki_roll"
  n-D Lookup Table/1 -> Saturation/1
  Tas/1 -> n-D Lookup Table/1
  Kp controllore beccheggio1/1 -> Bus Creator1/1  "Kp_becch"
  Ki controllore  beccheggio1/1 -> Bus Creator1/2  "Ki_becch"
  Kp controllore velocità beccheggio1/1 -> Bus Creator1/3  "Kp_q"
  K controllo imbardata inversa/1 -> Bus Creator1/19  "K_imb_inv"

== system autopilota_v_15_last/Subsystem1 ==
  note: MODI A/P
  note: LOOP ESTERNI e SWITCH
  note: LOOP INTERNI e SWITCH
  note: SISTEMA DI GESTIONE
  Comandi Manuali : Inport
  "Interruttori " : Inport  Port=2
  Riferimenti : Inport  Port=3
  Parametri Sistema di Controllo : Inport  Port=4
  SENSORI : Inport  Port=5
  int_sw_safe_interv : Inport  Port=6
  Cal_home : Inport  Port=7
  AUTOPILOTI1 : Subsystem
  CONTROLLI INTERNI E SWITCH1 : Subsystem
  Demux : Demux  Outputs=2
  GESTIONE AUTOPILOTI1 : Subsystem
  Mux : Mux  Inputs=2
  Mux1 : Mux  Inputs=3
  Subsystem1 : Subsystem
  COMANDI ATTUATORI : Outport  VectorParamsAs1DForOutWhenUnconnected=off
  AP_Alarm : Outport  Port=2  VectorParamsAs1DForOutWhenUnconnected=off
  H_LAT : Outport  Port=3  VectorParamsAs1DForOutWhenUnconnected=off
  H_LONG : Outport  Port=4  VectorParamsAs1DForOutWhenUnconnected=off
  H_ALT : Outport  Port=5  VectorParamsAs1DForOutWhenUnconnected=off
  Riferimenti Carrello : Outport  Port=6  VectorParamsAs1DForOutWhenUnconnected=off
  wires:
  Subsystem1/2(Inner_loop_ATO) -> CONTROLLI INTERNI E SWITCH1/10(Inner_loop_ATO)
  Subsystem1/5(H_ALT) -> H_ALT/1
  [Switch_AL] -> CONTROLLI INTERNI E SWITCH1/8(Switch_AL)
  [Switch_ATO] -> CONTROLLI INTERNI E SWITCH1/7(Switch_ATO)
  Parametri Sistema di Controllo/1 -> CONTROLLI INTERNI E SWITCH1/1(Parametri Sistema di Controllo), AUTOPILOTI1/2(Parametri Sistema di Controllo)
  CONTROLLI INTERNI E SWITCH1/2(theta_track) -> AUTOPILOTI1/10(traking theta)
  Subsystem1/3(H_LAT) -> H_LAT/1
  Subsystem1/4(H_LONG) -> H_LONG/1
  CONTROLLI INTERNI E SWITCH1/1(Comandi Attuatori) -> COMANDI ATTUATORI/1
  Comandi Manuali/1 -> CONTROLLI INTERNI E SWITCH1/2(Comandi Manuali), AUTOPILOTI1/6(comandi), GESTIONE AUTOPILOTI1/3(Comandi Manuali)
  AUTOPILOTI1/2(Riferimenti Rollio e Beccheggio) -> CONTROLLI INTERNI E SWITCH1/6(Riferimenti Rollio e Beccheggio)
  GESTIONE AUTOPILOTI1/5(Alarm Safe) -> AUTOPILOTI1/5(Alarm Safe), Mux/1
  Cal_home/1 -> Subsystem1/5(Cal_Home)
  GESTIONE AUTOPILOTI1/1(Switch Attuatori) -> Subsystem1/6(Switch_attuatori), CONTROLLI INTERNI E SWITCH1/4(Switch Attuatori), AUTOPILOTI1/7(Switch attuatori)
  Demux/1 -> GESTIONE AUTOPILOTI1/4(int_sw_safe)
  Demux/2 -> GESTIONE AUTOPILOTI1/5(int_sw_intervento)
  GESTIONE AUTOPILOTI1/4(Alarm Intervento) -> Mux/2
  Riferimenti/1 -> Subsystem1/3(waypoints e riferimenti vettoriali)
  GESTIONE AUTOPILOTI1/2(Riferimenti Safe) -> AUTOPILOTI1/4(Riferimenti Safe)
  SENSORI/1 -> GESTIONE AUTOPILOTI1/1(Sensori), Subsystem1/1(sensori), CONTROLLI INTERNI E SWITCH1/5(Sensori), AUTOPILOTI1/1(Sensori)
  Subsystem1/1(Riferimenti) -> CONTROLLI INTERNI E SWITCH1/9(riferimenti), AUTOPILOTI1/3(Riferimenti)
  GESTIONE AUTOPILOTI1/3(modo) -> Subsystem1/4(modo)
  int_sw_safe_interv/1 -> Demux/1
  [Switch_ATO] -> AUTOPILOTI1/8(Switch_ATO)
  GESTIONE AUTOPILOTI1/7(Switch_AL) -> [Switch_AL]
  AUTOPILOTI1/1(Riferimento Manetta) -> CONTROLLI INTERNI E SWITCH1/3(Riferimento Manetta)
  "Interruttori "/1 -> Subsystem1/2(Interruttori), GESTIONE AUTOPILOTI1/2("Interruttori ")
  Mux/1 -> AP_Alarm/1
  GESTIONE AUTOPILOTI1/6(Switch_ATO) -> [Switch_ATO]
  [Switch_AL] -> AUTOPILOTI1/9(Switch_AL)
  CONTROLLI INTERNI E SWITCH1/3(manetta_track) -> AUTOPILOTI1/11(manetta_track)
  CONTROLLI INTERNI E SWITCH1/4(track_phi) -> AUTOPILOTI1/12(track_phi)
  [Fase_ATO] -> Mux1/2  "Fase_ATO"
  Mux1/1 -> Riferimenti Carrello/1
  [modo] -> Mux1/1  "modo"
  [selector_AL] -> Mux1/3  "selector_AL"

== system autopilota_v_15_last/scalature comandi  ==
  note: 02/01/2022
      |
      | Abbiamo inserito un blocco "Cast to double"
      | dentro i blocchi: "THROTTLE1", "ELEVATOR1"
      | "AILERON1", ""RUDDER6"
  In1 : Inport
  AILERON1 : Subsystem
  Bus Creator : BusCreator  Inputs=4  OutDataTypeStr=Bus: slBus8_comandi
  Bus Selector : BusSelector  OutputSignals=Manetta,Equilibratore,Alettoni,Timone
  ELEVATOR1 : Subsystem
  RUDDER6 : Subsystem
  Radians to Degrees : simulink_extras/Transformations/Radians to Degrees
  Radians to Degrees1 : simulink_extras/Transformations/Radians to Degrees
  Radians to Degrees2 : simulink_extras/Transformations/Radians to Degrees
  THROTTLE1 : Subsystem
  Out1 : Outport  OutDataTypeStr=Bus: slBus8_comandi  VectorParamsAs1DForOutWhenUnconnected=off
  wires:
  Bus Creator/1 -> Out1/1
  ELEVATOR1/1(Out1) -> Bus Creator/2  "Equilibratore"
  RUDDER6/1(Out1) -> Bus Creator/4  "Timone"
  Bus Selector/4 -> Radians to Degrees2/1  "<Timone>"
  Bus Selector/1 -> THROTTLE1/1(In1)  "<Manetta>"
  Bus Selector/2 -> Radians to Degrees/1  "<Equilibratore>"
  Bus Selector/3 -> Radians to Degrees1/1  "<Alettoni>"
  THROTTLE1/1(Out1) -> Bus Creator/1  "Manetta"
  AILERON1/1(Out1) -> Bus Creator/3  "Alettoni"
  Radians to Degrees/1 -> ELEVATOR1/1(In1)
  Radians to Degrees1/1 -> AILERON1/1(In1)
  Radians to Degrees2/1 -> RUDDER6/1(In1)
  In1/1 -> Bus Selector/1

== system autopilota_v_15_last/MISURE DA SENSORI FILTRATE/AOA1 ==
  theta : Inport
  Tas : Inport  Port=2
  RC : Inport  Port=3
  Divide : Product  Inputs=*/
  Sum1 : Sum  Inputs=+-|
  Trigonometric Function : Trigonometry  Operator=asin
  AOA : Outport  VectorParamsAs1DForOutWhenUnconnected=off
  wires:
  RC/1 -> Divide/1
  Trigonometric Function/1 -> Sum1/2
  Tas/1 -> Divide/2
  Sum1/1 -> AOA/1
  Divide/1 -> Trigonometric Function/1
  theta/1 -> Sum1/1

== system autopilota_v_15_last/MISURE DA SENSORI FILTRATE/AOA2 ==
  theta : Inport
  Tas : Inport  Port=2
  RC : Inport  Port=3
  Divide : Product  Inputs=*/
  Sum1 : Sum  Inputs=+-|
  Trigonometric Function : Trigonometry  Operator=asin
  AOA : Outport  VectorParamsAs1DForOutWhenUnconnected=off
  wires:
  RC/1 -> Divide/1
  Trigonometric Function/1 -> Sum1/2
  Tas/1 -> Divide/2
  Sum1/1 -> AOA/1
  Divide/1 -> Trigonometric Function/1
  theta/1 -> Sum1/1

== system autopilota_v_15_last/MISURE DA SENSORI FILTRATE/Filter1B ==
  Misure : Inport
  Cond_ini : Inport  Port=2
  Q : Inport  Port=3
  R : Inport  Port=4
  sensors offset : Inport  Port=5
  Clock_gps_pos : Inport  Port=6
  Clock_gps_vel : Inport  Port=7
  Clock_mti : Inport  Port=8
  update : Inport  Port=9
  k_update : Inport  Port=10
  Enable : EnablePort
  DEFINITIVA : MATLAB Function  TreatAsAtomicUnit=on
  Lat : Outport  VectorParamsAs1DForOutWhenUnconnected=off
  Long : Outport  Port=2  VectorParamsAs1DForOutWhenUnconnected=off
  h : Outport  Port=3  VectorParamsAs1DForOutWhenUnconnected=off
  vn : Outport  Port=4  VectorParamsAs1DForOutWhenUnconnected=off
  ve : Outport  Port=5  VectorParamsAs1DForOutWhenUnconnected=off
  vd : Outport  Port=6  VectorParamsAs1DForOutWhenUnconnected=off
  an : Outport  Port=7  VectorParamsAs1DForOutWhenUnconnected=off
  ae : Outport  Port=8  VectorParamsAs1DForOutWhenUnconnected=off
  ad : Outport  Port=9  VectorParamsAs1DForOutWhenUnconnected=off
  p : Outport  Port=10  VectorParamsAs1DForOutWhenUnconnected=off
  q : Outport  Port=11  VectorParamsAs1DForOutWhenUnconnected=off
  r : Outport  Port=12  VectorParamsAs1DForOutWhenUnconnected=off
  bax : Outport  Port=13  VectorParamsAs1DForOutWhenUnconnected=off
  bay : Outport  Port=14  VectorParamsAs1DForOutWhenUnconnected=off
  baz : Outport  Port=15  VectorParamsAs1DForOutWhenUnconnected=off
  bp : Outport  Port=16  VectorParamsAs1DForOutWhenUnconnected=off
  bq : Outport  Port=17  VectorParamsAs1DForOutWhenUnconnected=off
  br : Outport  Port=18  VectorParamsAs1DForOutWhenUnconnected=off
  V_k : Outport  Port=19  VectorParamsAs1DForOutWhenUnconnected=off
  Imbardata : Outport  Port=20  VectorParamsAs1DForOutWhenUnconnected=off
  residui : Outport  Port=21  VectorParamsAs1DForOutWhenUnconnected=off
  Cov_est : Outport  Port=22  VectorParamsAs1DForOutWhenUnconnected=off
  wires:
  update/1 -> DEFINITIVA/9(update)
  Clock_mti/1 -> DEFINITIVA/8(clock_MTi)
  Clock_gps_vel/1 -> DEFINITIVA/7(clock_GPS_vel)
  sensors offset/1 -> DEFINITIVA/5(Sensor_Offsets)
  DEFINITIVA/5(ve_K) -> ve/1
  R/1 -> DEFINITIVA/4(R)
  Misure/1 -> DEFINITIVA/1(Misure)
  DEFINITIVA/2(Long_K) -> Long/1
  DEFINITIVA/1(Lat_K) -> Lat/1
  DEFINITIVA/4(vn_K) -> vn/1
  DEFINITIVA/3(h_K) -> h/1
  Q/1 -> DEFINITIVA/3(Q)
  DEFINITIVA/6(vd_K) -> vd/1
  Cond_ini/1 -> DEFINITIVA/2(x_prd_ini)
  Clock_gps_pos/1 -> DEFINITIVA/6(clock_GPS_pos)
  DEFINITIVA/7(an_K) -> an/1
  DEFINITIVA/8(ae_K) -> ae/1
  DEFINITIVA/9(ad_K) -> ad/1
  DEFINITIVA/10(p_K) -> p/1
  DEFINITIVA/11(q_K) -> q/1
  DEFINITIVA/12(r_K) -> r/1
  DEFINITIVA/13(baccx) -> bax/1
  DEFINITIVA/14(baccy) -> bay/1
  DEFINITIVA/15(baccz) -> baz/1
  DEFINITIVA/16(bp) -> bp/1
  DEFINITIVA/17(bq) -> bq/1
  DEFINITIVA/18(br) -> br/1
  DEFINITIVA/19(v_K) -> V_k/1
  DEFINITIVA/20(imbardata) -> Imbardata/1
  DEFINITIVA/21(residui) -> residui/1
  DEFINITIVA/22(Cov_est) -> Cov_est/1
  k_update/1 -> DEFINITIVA/10(k_update)

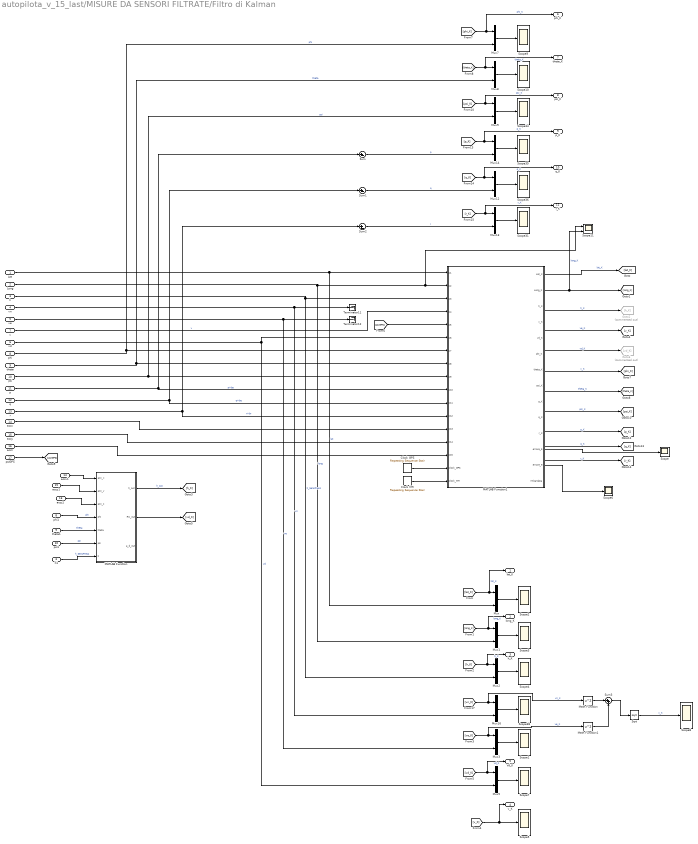
== system autopilota_v_15_last/MISURE DA SENSORI FILTRATE/Filtro di Kalman ==
  "Lat " : Inport
  "Long " : Inport  Port=2
  h : Inport  Port=3
  vn : Inport  Port=4
  "ve " : Inport  Port=5
  vd : Inport  Port=6
  "v " : Inport  Port=7
  phi : Inport  Port=8
  theta : Inport  Port=9
  psi : Inport  Port=10
  p : Inport  Port=11
  q : Inport  Port=12
  r : Inport  Port=13
  accx : Inport  Port=14
  accy : Inport  Port=15
  accz : Inport  Port=16
  psiGPS : Inport  Port=17
  Clock GPS : simulink/Sources/Repeating Sequence Stair  OutValues=[1 0 0 0 0 0 0 0 0 0 0 0 0 0 0 0 0 0 0 0 0 0 0 0 0 0 0 0 0 0 0 0 0 0 0 0 0 0 0 0 0 0 0 0 0 0 0 0 0 0]  tsamp=0.02  OutMin=[]  OutMax=[]  OutDataTypeStr=double  OutputDataTypeScalingMode=double  OutDataType=fixdt(0,8)  ConRadixGroup=Best Precision: Vector-wise  OutScaling=2^-12
  Clock MTi : simulink/Sources/Repeating Sequence Stair  OutValues=[1 0 1 0 1 0 1 0 1 0 1 0 1 0 1 0 1 0 1 0 1 0 1 0 1 0 1 0 1 0 1 0 1 0 1 0 1 0 1 0 1 0 1 0 1 0 1 0 1 0 ]  tsamp=0.02  OutMin=[]  OutMax=[]  OutDataTypeStr=double  OutputDataTypeScalingMode=double  OutDataType=fixdt(0,8)  ConRadixGroup=Best Precision: Vector-wise  OutScaling=2^-12
  Goto2 : Goto  Commented=on  GotoTag=h_K
  Goto6 : Goto  Commented=on  GotoTag=vd_K
  MATLAB Function : MATLAB Function  TreatAsAtomicUnit=on
  MATLAB Function1 : MATLAB Function  TreatAsAtomicUnit=on
  Math Function : Math  Operator=square  SignedPower=on  SaturateOnIntegerOverflow=on
  Math Function1 : Math  Operator=square  SignedPower=on  SaturateOnIntegerOverflow=on
  Mux{,1..3,5,7..9,12..14,16} (12 alike) : Mux  Inputs=2
  Scope{,1..10,31,34..36,38} (16 alike) : Scope
  Scope11 : Scope  NumInputPorts=2
  Sqrt : Sqrt  SaturateOnIntegerOverflow=on
  Sum : Sum  Inputs=|+-
  Sum1 : Sum  Inputs=|+-
  Sum2 : Sum  Inputs=|+-
  Sum3 : Sum  Inputs=|++
  Terminator11 : Terminator
  Terminator12 : Terminator
  accx1 : InportShadow  Port=14
  accy1 : InportShadow  Port=15
  accz1 : InportShadow  Port=16
  h1 : InportShadow  Port=3
  phi1 : InportShadow  Port=8
  psi1 : InportShadow  Port=10
  theta1 : InportShadow  Port=9
  lat_K : Outport  VectorParamsAs1DForOutWhenUnconnected=off
  long_K : Outport  Port=2  VectorParamsAs1DForOutWhenUnconnected=off
  h_K : Outport  Port=3  VectorParamsAs1DForOutWhenUnconnected=off
  v_K : Outport  Port=4  VectorParamsAs1DForOutWhenUnconnected=off
  Vd_K : Outport  Port=5  VectorParamsAs1DForOutWhenUnconnected=off
  phi_K : Outport  Port=6  VectorParamsAs1DForOutWhenUnconnected=off
  theta_K : Outport  Port=7  VectorParamsAs1DForOutWhenUnconnected=off
  psi_K : Outport  Port=8  VectorParamsAs1DForOutWhenUnconnected=off
  p_K : Outport  Port=9  VectorParamsAs1DForOutWhenUnconnected=off
  q_K : Outport  Port=10  VectorParamsAs1DForOutWhenUnconnected=off
  r_K : Outport  Port=11  VectorParamsAs1DForOutWhenUnconnected=off
  wires:
  MATLAB Function1/1(Lat_K) -> [lat_K]  "lat_K"
  MATLAB Function1/2(Long_K) -> Scope11/2, [long_K]  "long_K"
  MATLAB Function1/3(h_K) -> Goto2/1  "h_K"
  MATLAB Function1/4(v_K) -> [v_K]  "ve_K"
  MATLAB Function1/5(vd_K) -> Goto6/1  "vd_K"
  "Lat "/1 -> MATLAB Function1/1(z1), Mux/2  "lat"
  [lat_K] -> lat_K/1, Mux/1  "lat_K"
  Mux1/1 -> Scope3/1
  "Long "/1 -> Scope11/1, MATLAB Function1/2(z2), Mux1/2  "long"
  [long_K] -> long_K/1, Mux1/1  "long_K"
  Mux2/1 -> Scope4/1
  [h_K] -> h_K/1, Mux2/1  "h_K"
  Mux5/1 -> Scope7/1
  [vd_K] -> Vd_K/1, Mux5/1  "vd_K"
  Mux7/1 -> Scope9/1
  Mux8/1 -> Scope10/1
  [phi_K] -> phi_K/1, Mux7/1  "phi_K"
  [theta_K] -> theta_K/1, Mux8/1  "theta_K"
  Mux9/1 -> Scope34/1
  [psi_K] -> psi_K/1, Mux9/1  "psi_K"
  Mux14/1 -> Scope35/1
  Mux12/1 -> Scope36/1
  [q_K] -> q_K/1, Mux12/1  "q_K"
  Mux13/1 -> Scope31/1
  [r_K] -> r_K/1, Mux13/1  "r_K"
  [p_K] -> p_K/1, Mux14/1  "p_K"
  h/1 -> MATLAB Function1/3(z3), Mux2/2  "h_SensPress"
  Mux16/1 -> Scope38/1
  [vn_K] -> Math Function/1, Mux16/1  "vn_K"
  vn/1 -> Terminator11/1, Mux16/2  "vn"
  Mux/1 -> Scope2/1
  accx/1 -> MATLAB Function1/13(z13)
  accz/1 -> MATLAB Function1/15(z15)
  accy/1 -> MATLAB Function1/14(z14)
  MATLAB Function1/7(theta_K) -> [theta_K]  "theta_K"
  MATLAB Function1/8(psi_K) -> [psi_K]  "psi_K"
  MATLAB Function1/10(q_K) -> [q_K]  "q_K"
  MATLAB Function1/11(r_K) -> [r_K]  "r_K"
  Mux3/1 -> Scope1/1
  [ve_K] -> Math Function1/1, Mux3/1  "ve_K"
  "ve "/1 -> Terminator12/1, Mux3/2  "ve"
  vd/1 -> MATLAB Function1/6(z6), Mux5/2  "vd"
  phi/1 -> MATLAB Function1/7(z7), Mux7/2  "phi"
  theta/1 -> MATLAB Function1/8(z8), Mux8/2  "theta"
  psi/1 -> MATLAB Function1/9(z9), Mux9/2  "psi"
  p/1 -> MATLAB Function1/10(z10), Sum/1  "p+bp"
  q/1 -> MATLAB Function1/11(z11), Sum1/1  "q+bq"
  Sum/1 -> Mux14/2  "p"
  Sum1/1 -> Mux12/2  "q"
  Sum2/1 -> Mux13/2  "r"
  r/1 -> MATLAB Function1/12(z12), Sum2/1  "r+br"
  psiGPS/1 -> [psiGPS]
  [psiGPS] -> MATLAB Function1/5(z5)
  MATLAB Function1/6(phi_K) -> [phi_K]  "v_K"
  MATLAB Function1/9(p_K) -> [p_K]  "p_K"
  "v "/1 -> MATLAB Function1/4(z4)  "v"
  Math Function/1 -> Sum3/1
  Math Function1/1 -> Sum3/2
  Sum3/1 -> Sqrt/1
  Sqrt/1 -> Scope8/1  "v_K"
  Clock MTi/1 -> MATLAB Function1/17(clock_MTi)
  Clock GPS/1 -> MATLAB Function1/16(clock_GPS)
  [v_K] -> v_K/1, Scope5/1
  MATLAB Function1/12(errore_5) -> Scope/1
  MATLAB Function1/13(errore_9) -> Scope6/1
  theta1/1 -> MATLAB Function/5(theta)  "theta"
  phi1/1 -> MATLAB Function/4(phi)  "phi"
  psi1/1 -> MATLAB Function/6(psi)  "psi"
  h1/1 -> MATLAB Function/7(h)  "h_SensPress"
  accz1/1 -> MATLAB Function/3(acc_z)
  accy1/1 -> MATLAB Function/2(acc_y)
  accx1/1 -> MATLAB Function/1(acc_x)
  MATLAB Function/1(h_out) -> [h_K]  "h_out"
  MATLAB Function/2(RC_out) -> [vd_K]

== system autopilota_v_15_last/MISURE DA SENSORI FILTRATE/MISURE1B ==
  In1 : Inport
  Demux1 : Demux  Outputs=15
  Mux3 : Mux  Inputs=14
  Terminator1 : Terminator
  Out1 : Outport  VectorParamsAs1DForOutWhenUnconnected=off
  wires:
  Demux1/11 -> Mux3/10
  Demux1/12 -> Mux3/11
  Demux1/8 -> Mux3/8
  Demux1/15 -> Mux3/14
  Demux1/7 -> Mux3/7
  Demux1/6 -> Mux3/6
  In1/1 -> Demux1/1
  Mux3/1 -> Out1/1
  Demux1/1 -> Mux3/1
  Demux1/2 -> Mux3/2
  Demux1/3 -> Mux3/3
  Demux1/4 -> Mux3/4
  Demux1/5 -> Mux3/5
  Demux1/10 -> Mux3/9
  Demux1/13 -> Mux3/12
  Demux1/14 -> Mux3/13
  Demux1/9 -> Terminator1/1  "psi corretta"

== system autopilota_v_15_last/MISURE DA SENSORI FILTRATE/Subsystem ==
  0-360 : Inport
  Constant : Constant  Value=360
  Sum : Sum  Inputs=|+-
  Switch : Switch  Criteria=u2 > Threshold  Threshold=180
  "+-180 " : Outport  VectorParamsAs1DForOutWhenUnconnected=off
  wires:
  0-360/1 -> Switch/2, Switch/3, Sum/1
  Sum/1 -> Switch/1
  Constant/1 -> Sum/2
  Switch/1 -> "+-180 "/1

== system autopilota_v_15_last/MISURE DA SENSORI FILTRATE/Subsystem2 ==
  +-180 : Inport
  Constant : Constant  Value=360
  Gain : Gain  Gain=-1
  Sum : Sum  Inputs=|++
  Switch : Switch  Criteria=u2 > Threshold
  0-360 : Outport  VectorParamsAs1DForOutWhenUnconnected=off
  wires:
  Switch/1 -> 0-360/1
  Sum/1 -> Switch/1
  Gain/1 -> Switch/2
  +-180/1 -> Sum/1, Switch/3, Gain/1
  Constant/1 -> Sum/2
